simulink model "TEST_2"  (R2024a)
settings: Solver=VariableStepAuto  StartTime=0.0  StopTime=1  RelTol=1e-3
values from neighbouring files (symbols this model uses):
  a = 1.3    [TEST.m]    (also in batter_y.m = -k_omega / J)
  autoRecharge = 0    [TEST.m]
  Cdc = 278e-3    (= 0.278)    [TEST.m]    (also in batter_y.m)
  Efficiency = 96    [TEST.m]
  fg = 60    [TEST.m]    (also in batter_y.m)
  Fn = 60    [TEST.m]
  Gn = 1000    [TEST.m]    (also in batter_y.m)
  Initial_kWh_pc = 80    [TEST.m]
  Ipv_n = Isc_n*(Rp+Rs)/Rp    (= 8.21426513558)    [TEST.m]    (also in batter_y.m)
  Isc_n = 8.21    [TEST.m]    (also in batter_y.m)
  k = 1.3806503e-23    [TEST.m]    (also in batter_y.m)
  KI = 0.0032    [TEST.m]    (also in batter_y.m)
  Ki_C = Rc/tau_C    (= 0.768)    [TEST.m]    (also in batter_y.m)
  Ki_DC = omega_DC^2*Cdc    [TEST.m]    (also in batter_y.m)
  Ki_P = 1/(Ki_pq*tau_P)    [TEST.m]    (also in batter_y.m)
  Ki_PLL = Kp_PLL/tau_PLL    [TEST.m]    (also in batter_y.m)
  Kp_C = Lc/tau_C    (= 0.020372)    [TEST.m]    (also in batter_y.m)
  Kp_DC = 2*xi_DC*omega_DC*Cdc    [TEST.m]    (also in batter_y.m)
  Kp_P = tau_C/(Ki_pq*tau_P)    [TEST.m]    (also in batter_y.m)
  Kp_PLL = xi_PLL*2*omega_PLL/Vp    [TEST.m]    (also in batter_y.m)
  KV = -0.123    [TEST.m]    (also in batter_y.m)
  KVmp = Vmp_n/Voc_n    (= 0.799392097264)    [TEST.m]    (also in batter_y.m)
  kWh_Rated = 100    [TEST.m]
  Lc = 20.372e-6    (= 2.0372e-05)    [TEST.m]    (also in batter_y.m)
  LowChrgLim = LimitVec(2)    [TEST.m]
  Np = 345    [TEST.m]    (also in batter_y.m)
  Ns = 45    [TEST.m]    (also in batter_y.m)
  Ns_cell = 54    [TEST.m]    (also in batter_y.m)
  Pnom = PnomkW*1e3    (= 500000)    [TEST.m]    (also in batter_y.m = 1500000)
  Precharge = 50    [TEST.m]
  q = 1.6021764e-19    [TEST.m]    (also in batter_y.m)
  Rc = 0.768e-3    (= 0.000768)    [TEST.m]    (also in batter_y.m)
  RechargeSOC = 11    [TEST.m]
  Rp = 425.405    [TEST.m]    (also in batter_y.m)
  Rs = 0.221    [TEST.m]    (also in batter_y.m)
  Tn = 25    [TEST.m]    (also in batter_y.m)
  UpChrgLim = LimitVec(1)    [TEST.m]
  Vdc = 1200    [TEST.m]    (also in batter_y.m)
  Vn = 4000    [TEST.m]
  Voc_n = 32.9    [TEST.m]    (also in batter_y.m)
  Vp = Ug*sqrt(2)/sqrt(3)    [TEST.m]    (also in batter_y.m)
libraries: spsSeriesRLCBranchLib x21, spsThreePhaseSeriesRLCLoadLib x7, simulink x6, spsSeriesRLCLoadLib x5, spsGroundLib x5, slpidlib x5, spsControlledVoltageSourceLib x3, spsThreePhaseVIMeasurementLib x2, spsCurrentMeasurementLib x2, spsControlledCurrentSourceLib x2, spsThreePhaseTransformerTwoWindingsLib x2, spsThreePhaseSourceLib x1
(part 1 of 2)
settings Model: Creator=Dell  LastModifiedBy=Dell

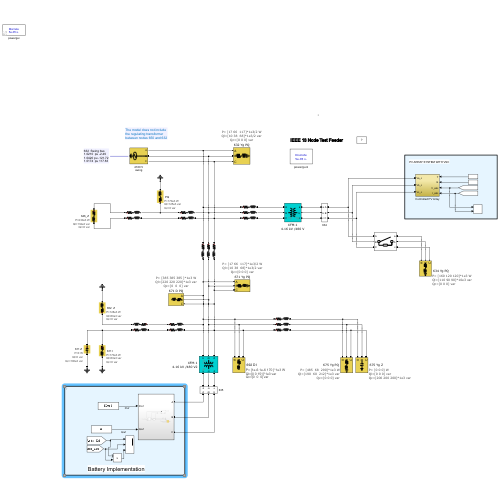
[thumbnail: Simulink's stored preview of the top-level diagram]
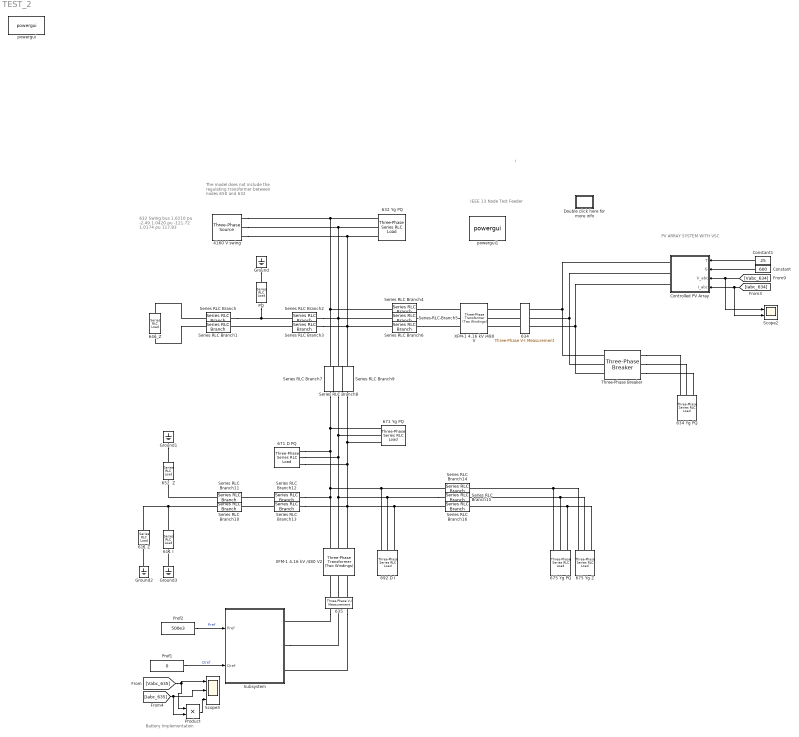
== system TEST_2 ==
  note: PV ARRAY SYSTEM WITH VSC
  note: 632 Swing bus
      | 1.0210 pu -2.49
      | 1.0420 pu -121.72
      | 1.0174 pu 117.83
  note: The model does not include
      | the regulating transformer
      | between nodes 650 and 632
  note: IEEE 13 Node Test Feeder
  note: i
  note: Battery Implementation
  " 634 Yg PQ " : spsThreePhaseSeriesRLCLoadLib/Three-Phase Series RLC Load  LConnTagsString=A|B|C  Configuration=Y (grounded)  NominalVoltage=120e3  Vabc=[ 0.993805 1.0218 0.995862]*277.128  Vabcp=[1e3 1e3 1e3]  NominalFrequency=60  UnbalancedPower=on  ActivePower=1e+006  InductivePower=0  CapacitivePower=0  Pabc=[160 120 120]*1e3  QLabc=[110 90 90]*10e3  QCabc=[0 0 0]  Pabcp=[10e3 9e3 11e3]  QLabcp=[100 90 110]  QCabcp=[100 90 110]  Measurements=None  LoadType=constant PQ
      settings: AttributesFormatString=|
      | P= %<Pabc> W
      | Ql=%<QLabc> var
      | Qc=%<QCabc> var
  4160 V swing : spsThreePhaseSourceLib/Three-Phase Source  InternalConnection=Yg  VoltagePhases=on  Voltage=4.16e3  PhaseAngle=0  Voltage_phases=[ 1.021 1.042 1.0174]*2401.78  PhaseAngles_phases=[ -2.49 -121.72 117.83]  Frequency=60  NonIdealSource=off  SpecifyImpedance=on  Resistance=0.8929  Inductance=16.58e-3  ShortCircuitLevel=100e6  BaseVoltage=120e3  XRratio=10  BusType=swing  Pref=0  Qref=0  Prefabc=[0 0 0]  Qrefabc=[0 0 0]  Qmin="[-inf  -inf -inf]"  Qmax="[inf  inf inf]"
  611 I : spsSeriesRLCLoadLib/Series RLC Load  LConnTagsString=a  RConnTagsString=__new0  NominalVoltage=0.986941*2401.78  NominalFrequency=60  ActivePower=170e3  InductivePower=80e3  CapacitivePower=0  Setx0=off  InitialVoltage=0  SetiL0=off  InitialCurrent=0  Measurements=Branch voltage and current  LoadType=constant I
      settings: AttributesFormatString=|
      | P=%<ActivePower> W
      | Ql=%<InductivePower> var
      | Qc=%<CapacitivePower> var
  611 Z : spsSeriesRLCLoadLib/Series RLC Load  LConnTagsString=a  RConnTagsString=__new0  NominalVoltage=4160/sqrt(3)  NominalFrequency=60  ActivePower=0  InductivePower=0  CapacitivePower=100e3  Setx0=off  InitialVoltage=0  SetiL0=off  InitialCurrent=0  Measurements=None  LoadType=constant Z
      settings: AttributesFormatString=|
      | P=%<ActivePower> W
      | Ql=%<InductivePower> var
      | Qc=%<CapacitivePower> var
  632 Yg PQ : spsThreePhaseSeriesRLCLoadLib/Three-Phase Series RLC Load  LConnTagsString=A|B|C  Configuration=Y (grounded)  NominalVoltage=120e3  Vabc=[ 1.021 1.042 1.0174]*2401.78  Vabcp=[1e3 1e3 1e3]  NominalFrequency=60  UnbalancedPower=on  ActivePower=1e+006  InductivePower=0  CapacitivePower=0  Pabc="[17 66  117]*1e3/2"  QLabc="[10 38  68]*1e3/2"  QCabc=[0 0 0]  Pabcp=[10e3 9e3 11e3]  QLabcp=[100 90 110]  QCabcp=[100 90 110]  Measurements=None  LoadType=constant PQ
      settings: AttributesFormatString=|
      | P= %<Pabc> W
      | Ql=%<QLabc> var
      | Qc=%<QCabc> var
  634 : spsThreePhaseVIMeasurementLib/Three-Phase V-I Measurement  VoltageMeasurement=phase-to-ground  SetLabelV=on  LabelV=Vabc_634  Vpu=off  VpuLL=off  CurrentMeasurement=yes  SetLabelI=on  LabelI=Iabc_634  Ipu=off  Pbase=100e6  Vbase=4160  OutputType=Complex  PhasorSimulation=off  PSBequivalent=0
  635 : spsThreePhaseVIMeasurementLib/Three-Phase V-I Measurement  VoltageMeasurement=phase-to-ground  SetLabelV=on  LabelV=Vabc_635  Vpu=off  VpuLL=off  CurrentMeasurement=yes  SetLabelI=on  LabelI=Iabc_635  Ipu=off  Pbase=100e6  Vbase=4160  OutputType=Complex  PhasorSimulation=off  PSBequivalent=0
  646_Z : spsSeriesRLCLoadLib/Series RLC Load  LConnTagsString=a  RConnTagsString=__new0  NominalVoltage=4160  NominalFrequency=60  ActivePower=230e3  InductivePower=132e3  CapacitivePower=0  Setx0=off  InitialVoltage=0  SetiL0=off  InitialCurrent=0  Measurements=None  LoadType=constant Z
      settings: AttributesFormatString=|
      | P=%<ActivePower> W
      | Ql=%<InductivePower> var
      | Qc=%<CapacitivePower> var
  "652  Z " : spsSeriesRLCLoadLib/Series RLC Load  LConnTagsString=a  RConnTagsString=__new0  NominalVoltage=4160/sqrt(3)  NominalFrequency=60  ActivePower=128e3  InductivePower=86e3  CapacitivePower=0  Setx0=off  InitialVoltage=0  SetiL0=off  InitialCurrent=0  Measurements=None  LoadType=constant Z
      settings: AttributesFormatString=|
      | P=%<ActivePower> W
      | Ql=%<InductivePower> var
      | Qc=%<CapacitivePower> var
  671 D PQ : spsThreePhaseSeriesRLCLoadLib/Three-Phase Series RLC Load  LConnTagsString=A|B|C  Configuration=Delta  NominalVoltage=120e3  Vabc="[1  1  1]*120e3/sqrt(3)"  Vabcp=[ 1.73773 1.77224 1.71484]*2401.78  NominalFrequency=60  UnbalancedPower=on  ActivePower=1e+006  InductivePower=0  CapacitivePower=0  Pabc="[17 66  117]*1e3/2"  QLabc="[10 38  68]*1e3/2"  QCabc=[0 0 0]  Pabcp=[385 385 385 ]*1e3  QLabcp=[220 220 220]*1e3  QCabcp="[0  0  0]"  Measurements=Branch voltages and currents  LoadType=constant PQ
      settings: AttributesFormatString=|
      | P= %<Pabcp> W
      | Ql=%<QLabcp> var
      | Qc=%<QCabcp> var
  671 Yg PQ : spsThreePhaseSeriesRLCLoadLib/Three-Phase Series RLC Load  LConnTagsString=A|B|C  Configuration=Y (grounded)  NominalVoltage=120e3  Vabc=[ 0.987076 1.0519 0.978043]*2401.78  Vabcp=[1e3 1e3 1e3]  NominalFrequency=60  UnbalancedPower=on  ActivePower=1e+006  InductivePower=0  CapacitivePower=0  Pabc="[17 66  117]*1e3/2"  QLabc="[10 38  68]*1e3/2"  QCabc=[0 0 0]  Pabcp=[10e3 9e3 11e3]  QLabcp=[100 90 110]  QCabcp=[100 90 110]  Measurements=None  LoadType=constant PQ
      settings: AttributesFormatString=|
      | P= %<Pabc> W
      | Ql=%<QLabc> var
      | Qc=%<QCabc> var
  675 Yg PQ : spsThreePhaseSeriesRLCLoadLib/Three-Phase Series RLC Load  LConnTagsString=A|B|C  Configuration=Y (grounded)  NominalVoltage=120e3  Vabc=[ 0.98063 1.05431 0.975983]*2401.78  Vabcp=[1e3 1e3 1e3]  NominalFrequency=60  UnbalancedPower=on  ActivePower=1e+006  InductivePower=0  CapacitivePower=0  Pabc="[485  68  290]*1e3"  QLabc="[190  60  212]*1e3"  QCabc=[0 0 0]  Pabcp=[10e3 9e3 11e3]  QLabcp=[100 90 110]  QCabcp=[100 90 110]  Measurements=Branch voltages and currents  LoadType=constant PQ
      settings: AttributesFormatString=|
      | P= %<Pabc> W
      | Ql=%<QLabc> var
      | Qc=%<QCabc> var
  675 Yg Z : spsThreePhaseSeriesRLCLoadLib/Three-Phase Series RLC Load  LConnTagsString=A|B|C  Configuration=Y (grounded)  NominalVoltage=120e3  Vabc="[1  1  1]*4160/sqrt(3)"  Vabcp=[1e3 1e3 1e3]  NominalFrequency=60  UnbalancedPower=on  ActivePower=1e+006  InductivePower=0  CapacitivePower=0  Pabc=[0 0 0]  QLabc=[0 0 0]  QCabc=[200 200 200]*1e3  Pabcp=[10e3 9e3 11e3]  QLabcp=[100 90 110]  QCabcp=[100 90 110]  Measurements=None  LoadType=constant Z
      settings: AttributesFormatString=|
      | P= %<Pabc> W
      | Ql=%<QLabc> var
      | Qc=%<QCabc> var
  692 D I : spsThreePhaseSeriesRLCLoadLib/Three-Phase Series RLC Load  LConnTagsString=A|B|C  Configuration=Delta  NominalVoltage=120e3  Vabc="[1  1  1]*120e3/sqrt(3)"  Vabcp=[ 1.73488 1.75203 1.72341]*2401.78  NominalFrequency=60  UnbalancedPower=on  ActivePower=1e+006  InductivePower=0  CapacitivePower=0  Pabc="[17 66  117]*1e3/2"  QLabc="[10 38  68]*1e3/2"  QCabc=[0 0 0]  Pabcp=[1e-6 1e-6 170 ]*1e3  QLabcp=[0 0 151]*1e3  QCabcp="[0  0  0]"  Measurements=Branch voltages and currents  LoadType=constant I
      settings: AttributesFormatString=|
      | P= %<Pabcp> W
      | Ql=%<QLabcp> var
      | Qc=%<QCabcp> var
  Constant : Constant  Value=600
  Constant1 : Constant  Value=25
  Controlled PV Array : Subsystem
      settings: PortSchema="{\"entries\":[{\"content\":{\"sides\":[{\"content\":{\"connectorIds\":[\"LConn1\",\"LConn2\",\"LConn3\"]},\"type\":\"ConnectorPlacement.EquallySpacedRectSide\",\"uuid\":\"92a05cf9-a19b-475d-bffb-9406018f82f4\"},{\"content\":{\"connectorIds\":[\"In1\",\"In2\",\"In3\",\"In4\"],\"side\":\"RIGHT\"},\"type\":\"ConnectorPlacement.EquallySpacedRectSide\",\"uuid\":\"83076eb6-0a86-49d7-8932-035501cdc6f6\"},{\"content\":{\"side\":\"TOP\"},\"type\":\"ConnectorPlacement.EquallySpacedRectSide\",\"uuid\":\"ba2310df-ee07-4a5c-88ff-ef0f81658322\"}]},\"type\":\"ConnectorPlacement.EquallySpacedConnector\",\"uuid\":\"9e64c472-0dae-4bb4-8eb3-3329c328d412\"}],\"packageUris\":[\"http://schema.mathworks.com/mf0/Connector/R2020b\"],\"version\":\"1.0\"}"
  Double click here for more info : Subsystem
      settings: OpenFcn=showdemo(bdroot(gcb))
      mask Display: disp('?')
  Ground{,1..3} (4 alike) : spsGroundLib/Ground  LConnTagsString=a
  PQ : spsSeriesRLCLoadLib/Series RLC Load  LConnTagsString=a  RConnTagsString=__new0  NominalVoltage=1.03289*2401.78  NominalFrequency=60  ActivePower=170e3  InductivePower=125e3  CapacitivePower=0  Setx0=off  InitialVoltage=0  SetiL0=off  InitialCurrent=0  Measurements=None  LoadType=constant PQ
      settings: AttributesFormatString=|
      | P=%<ActivePower> W
      | Ql=%<InductivePower> var
      | Qc=%<CapacitivePower> var
  Pref1 : Constant  Value=0
  Pref2 : Constant  Value=500e3
  Product : Product
  Scope2 : Scope  NumInputPorts=2
  Scope3 : Scope  NumInputPorts=3
  Series RLC Branch : spsSeriesRLCBranchLib/Series RLC Branch  LConnTagsString=__new0  RConnTagsString=__new0  BranchType=RL  Resistance=0.07553  Inductance=0.20302e-3  SetiL0=off  InitialCurrent=0  Capacitance=1e-6  Setx0=off  InitialVoltage=0  Measurements=None
  Series RLC Branch1 : spsSeriesRLCBranchLib/Series RLC Branch  LConnTagsString=__new0  RConnTagsString=__new0  BranchType=RL  Resistance=0.07553  Inductance=0.20302e-3  SetiL0=off  InitialCurrent=0  Capacitance=1e-6  Setx0=off  InitialVoltage=0  Measurements=None
  Series RLC Branch10 : spsSeriesRLCBranchLib/Series RLC Branch  LConnTagsString=__new0  RConnTagsString=__new0  BranchType=RL  Resistance=0.07552  Inductance=0.20308e-3  SetiL0=off  InitialCurrent=0  Capacitance=1e-6  Setx0=off  InitialVoltage=0  Measurements=None
  Series RLC Branch11 : spsSeriesRLCBranchLib/Series RLC Branch  LConnTagsString=__new0  RConnTagsString=__new0  BranchType=RL  Resistance=0.20340  Inductance=0.20593e-3  SetiL0=off  InitialCurrent=0  Capacitance=1e-6  Setx0=off  InitialVoltage=0  Measurements=None
  Series RLC Branch12 : spsSeriesRLCBranchLib/Series RLC Branch  LConnTagsString=__new0  RConnTagsString=__new0  BranchType=RL  Resistance=0.07521  Inductance=0.20450e-3  SetiL0=off  InitialCurrent=0  Capacitance=1e-6  Setx0=off  InitialVoltage=0  Measurements=None
  Series RLC Branch13 : spsSeriesRLCBranchLib/Series RLC Branch  LConnTagsString=__new0  RConnTagsString=__new0  BranchType=RL  Resistance=0.07521  Inductance=0.20450e-3  SetiL0=off  InitialCurrent=0  Capacitance=1e-6  Setx0=off  InitialVoltage=0  Measurements=None
  Series RLC Branch14 : spsSeriesRLCBranchLib/Series RLC Branch  LConnTagsString=__new0  RConnTagsString=__new0  BranchType=RL  Resistance=0.07559  Inductance=0.11210e-3  SetiL0=off  InitialCurrent=0  Capacitance=1e-6  Setx0=off  InitialVoltage=0  Measurements=None
  Series RLC Branch15 : spsSeriesRLCBranchLib/Series RLC Branch  LConnTagsString=__new0  RConnTagsString=__new0  BranchType=RL  Resistance=0.07559  Inductance=0.11210e-3  SetiL0=off  InitialCurrent=0  Capacitance=1e-6  Setx0=off  InitialVoltage=0  Measurements=None
  Series RLC Branch16 : spsSeriesRLCBranchLib/Series RLC Branch  LConnTagsString=__new0  RConnTagsString=__new0  BranchType=RL  Resistance=0.07559  Inductance=0.11210e-3  SetiL0=off  InitialCurrent=0  Capacitance=1e-6  Setx0=off  InitialVoltage=0  Measurements=None
  Series RLC Branch2 : spsSeriesRLCBranchLib/Series RLC Branch  LConnTagsString=__new0  RConnTagsString=__new0  BranchType=RL  Resistance=0.12589  Inductance=0.33837e-3  SetiL0=off  InitialCurrent=0  Capacitance=1e-6  Setx0=off  InitialVoltage=0  Measurements=None
  Series RLC Branch3 : spsSeriesRLCBranchLib/Series RLC Branch  LConnTagsString=__new0  RConnTagsString=__new0  BranchType=RL  Resistance=0.12589  Inductance=0.33837e-3  SetiL0=off  InitialCurrent=0  Capacitance=1e-6  Setx0=off  InitialVoltage=0  Measurements=None
  Series RLC Branch4 : spsSeriesRLCBranchLib/Series RLC Branch  LConnTagsString=__new0  RConnTagsString=__new0  BranchType=RL  Resistance=0.07126  Inductance=0.29675e-3  SetiL0=off  InitialCurrent=0  Capacitance=1e-6  Setx0=off  InitialVoltage=0  Measurements=None
  Series RLC Branch5 : spsSeriesRLCBranchLib/Series RLC Branch  LConnTagsString=__new0  RConnTagsString=__new0  BranchType=RL  Resistance=0.07126  Inductance=0.29675e-3  SetiL0=off  InitialCurrent=0  Capacitance=1e-6  Setx0=off  InitialVoltage=0  Measurements=None
  Series RLC Branch6 : spsSeriesRLCBranchLib/Series RLC Branch  LConnTagsString=__new0  RConnTagsString=__new0  BranchType=RL  Resistance=0.07126  Inductance=0.29675e-3  SetiL0=off  InitialCurrent=0  Capacitance=1e-6  Setx0=off  InitialVoltage=0  Measurements=None
  Series RLC Branch7 : spsSeriesRLCBranchLib/Series RLC Branch  LConnTagsString=__new0  RConnTagsString=__new0  BranchType=RL  Resistance=0.13124  Inductance=1.03632e-3  SetiL0=off  InitialCurrent=0  Capacitance=1e-6  Setx0=off  InitialVoltage=0  Measurements=None
  Series RLC Branch8 : spsSeriesRLCBranchLib/Series RLC Branch  LConnTagsString=__new0  RConnTagsString=__new0  BranchType=RL  Resistance=0.13124  Inductance=1.03632e-3  SetiL0=off  InitialCurrent=0  Capacitance=1e-6  Setx0=off  InitialVoltage=0  Measurements=None
  Series RLC Branch9 : spsSeriesRLCBranchLib/Series RLC Branch  LConnTagsString=__new0  RConnTagsString=__new0  BranchType=RL  Resistance=0.13124  Inductance=1.03632e-3  SetiL0=off  InitialCurrent=0  Capacitance=1e-6  Setx0=off  InitialVoltage=0  Measurements=None
  Subsystem : Subsystem
  Three-Phase Breaker : spsThreePhaseBreakerLib/Three-Phase Breaker  InitialState=open  SwitchA=on  SwitchB=on  SwitchC=on  SwitchTimes=0.3  External=off  BreakerResistance=0.01  SnubberResistance=1e6  SnubberCapacitance=inf  Measurements=None
  XFM-1 4.16 kV /480 V : spsThreePhaseTransformerTwoWindingsLib/Three-Phase Transformer (Two Windings)  Winding1Connection=Yg  Winding2Connection=Yg  CoreType=Three single-phase transformers  SetSaturation=off  Hysteresis=off  DataFile='hysteresis'  SetInitialFlux=off  Measurements=None  UNITS=pu  NominalPower=[ 500e3 , 60 ]  Winding1=[4160 0.011 0.02]  Winding2=[480 0 0]  Rm=500  Lm=500  L0=0.5  Saturation=[0 0;0.0024 1.2;1 1.52]  InitialFluxes=[0.8 -0.8 0.7]  BreakLoop=off  DiscreteSolver=Trapezoidal iterative  DataType=off  TransfoNumber=1
  XFM-1 4.16 kV /480 V2 : spsThreePhaseTransformerTwoWindingsLib/Three-Phase Transformer (Two Windings)  Winding1Connection=Yg  Winding2Connection=Yg  CoreType=Three single-phase transformers  SetSaturation=off  Hysteresis=off  DataFile='hysteresis'  SetInitialFlux=off  Measurements=None  UNITS=pu  NominalPower=[ 500e3 , 60 ]  Winding1=[4160 0.011 0.02]  Winding2=[480 0 0]  Rm=500  Lm=500  L0=0.5  Saturation=[0 0;0.0024 1.2;1 1.52]  InitialFluxes=[0.8 -0.8 0.7]  BreakLoop=off  DiscreteSolver=Trapezoidal iterative  DataType=off  TransfoNumber=1
  powergui : sps_lib/powergui  Priority=1  SimulationMode=Discrete  SampleTime=50e-6  frequency=60  Iterations=50  frequencyindice=0  Pbase=100e6  ErrMax=1e-4  UnitsV=kV  UnitsW=MW  buscounter=0  FunctionMessages=off  echomessages=off  EnableUseOfTLC=off  CurrentSourceSwitches=off  DisableSnubberDevices=off  DisableRonSwitches=off  DisableVfSwitches=off  DisplayEquations=off  AutomaticDiscreteSolvers=off  SolverType=Tustin/Backward Euler (TBE)  Interpol=off  ExternalGateDelay=off  methode=off  Ts=100  x0status=blocks  SPID=on  SwTol=0  HookPort=off  NonlinearTolerance=1e-4  nMaxIteration=100  ContinueOnMaxIteration=off  RestoreLinks=warning  ResistiveCurrentMeasurement=off  Frange=[0:2:500]  Ylog=off  Xlog=on  ShowGrid=off  save=off  variable=ZData  structure=0  ZoomFFT=off  StartTime=0.0  cycles=1  DisplayStyle=1  fundamental=60  FreqAxis=off  MaxFrequency=1000  frequencyindicesteady=1  RmsSteady=1  display=off
  powergui1 : spspowerguiLib/powergui  Priority=1  SimulationMode=Discrete  SampleTime=5e-5  frequency=60  Iterations=50  frequencyindice=0  Pbase=100e3  ErrMax=0.0001  UnitsV=kV  UnitsW=kW  buscounter=0  FunctionMessages=off  echomessages=off  EnableUseOfTLC=off  CurrentSourceSwitches=off  DisableSnubberDevices=off  DisableRonSwitches=off  DisableVfSwitches=off  DisplayEquations=off  AutomaticDiscreteSolvers=off  SolverType=Tustin/Backward Euler (TBE)  Interpol=off  ExternalGateDelay=off  methode=off  Ts=0  x0status=blocks  SPID=off  SwTol=0  HookPort=off  NonlinearTolerance=1e-4  nMaxIteration=100  ContinueOnMaxIteration=off  RestoreLinks=warning  ResistiveCurrentMeasurement=off  Frange=[0:2:500]  Ylog=off  Xlog=on  ShowGrid=off  save=off  variable=ZData  structure=0  ZoomFFT=on  StartTime=0.0  cycles=1  DisplayStyle=1  fundamental=60  FreqAxis=off  MaxFrequency=1000  frequencyindicesteady=1  RmsSteady=1  display=off
  wires:
  [Iabc_634] -> Scope2/2, Controlled PV Array/4(I_abc)
  Pref2/1 -> Subsystem/1(Pref)  "Pref"
  [Iabc_635] -> Product/2, Scope3/2
  [Vabc_634] -> Scope2/1, Controlled PV Array/3(V_abc)
  [Vabc_635] -> Product/1, Scope3/1
  Constant/1 -> Controlled PV Array/2(G)
  Pref1/1 -> Subsystem/2(Qref)  "Qref"
  Constant1/1 -> Controlled PV Array/1(T)
  Product/1 -> Scope3/3
  connections:
  Series RLC Branch5/LConn1 -- Series RLC Branch2/RConn1 -- 632 Yg PQ/LConn2 -- 4160 V swing/RConn2 -- Series RLC Branch8/LConn1
  XFM-1 4.16 kV /480 V2/LConn3 -- Series RLC Branch12/RConn1 -- 692 D I/LConn1 -- Series RLC Branch14/LConn1 -- 671 D PQ/LConn1 -- Series RLC Branch7/RConn1 -- 671 Yg PQ/LConn1
  Series RLC Branch2/LConn1 -- Series RLC Branch/RConn1 -- PQ/LConn1
  675 Yg PQ/LConn1 -- Series RLC Branch14/RConn1 -- 675 Yg Z/LConn1
  Three-Phase Breaker/LConn2 -- 634/LConn2 -- Controlled PV Array/LConn2
  Series RLC Branch6/LConn1 -- Series RLC Branch3/RConn1 -- 632 Yg PQ/LConn3 -- 4160 V swing/RConn3 -- Series RLC Branch9/LConn1
  675 Yg PQ/LConn3 -- Series RLC Branch16/RConn1 -- 675 Yg Z/LConn3
  Series RLC Branch15/LConn1 -- 671 D PQ/LConn2 -- Series RLC Branch8/RConn1 -- 671 Yg PQ/LConn2 -- XFM-1 4.16 kV /480 V2/LConn2 -- 692 D I/LConn2
  675 Yg PQ/LConn2 -- Series RLC Branch15/RConn1 -- 675 Yg Z/LConn2
  671 Yg PQ/LConn3 -- Series RLC Branch9/RConn1 -- Series RLC Branch13/RConn1 -- XFM-1 4.16 kV /480 V2/LConn1 -- 692 D I/LConn3 -- Series RLC Branch16/LConn1 -- 671 D PQ/LConn3
  Three-Phase Breaker/LConn3 -- 634/LConn3 -- Controlled PV Array/LConn3
  4160 V swing/RConn1 -- 632 Yg PQ/LConn1 -- Series RLC Branch4/LConn1 -- Series RLC Branch7/LConn1
  Series RLC Branch10/LConn1 -- 611 Z/LConn1 -- 611 I/LConn1
  Three-Phase Breaker/LConn1 -- 634/LConn1 -- Controlled PV Array/LConn1
  635/LConn3 -- Subsystem/RConn3
  Subsystem/RConn2 -- 635/LConn2
  Series RLC Branch3/LConn1 -- Series RLC Branch1/RConn1
  Ground/LConn1 -- PQ/RConn1
  Series RLC Branch11/RConn1 -- "652  Z "/LConn1
  635/LConn1 -- Subsystem/RConn1
  Series RLC Branch1/LConn1 -- 646_Z/RConn1
  Ground3/LConn1 -- 611 I/RConn1
  634/RConn1 -- XFM-1 4.16 kV /480 V/RConn1
  Ground2/LConn1 -- 611 Z/RConn1
  634/RConn2 -- XFM-1 4.16 kV /480 V/RConn2
  Series RLC Branch/LConn1 -- 646_Z/LConn1
  Ground1/LConn1 -- "652  Z "/RConn1
  635/RConn1 -- XFM-1 4.16 kV /480 V2/RConn3
  Series RLC Branch12/LConn1 -- Series RLC Branch11/LConn1
  Series RLC Branch5/RConn1 -- XFM-1 4.16 kV /480 V/LConn2
  XFM-1 4.16 kV /480 V/LConn3 -- Series RLC Branch6/RConn1
  635/RConn3 -- XFM-1 4.16 kV /480 V2/RConn1
  Three-Phase Breaker/RConn2 -- " 634 Yg PQ "/LConn2
  635/RConn2 -- XFM-1 4.16 kV /480 V2/RConn2
  634/RConn3 -- XFM-1 4.16 kV /480 V/RConn3
  XFM-1 4.16 kV /480 V/LConn1 -- Series RLC Branch4/RConn1
  Three-Phase Breaker/RConn3 -- " 634 Yg PQ "/LConn3
  Three-Phase Breaker/RConn1 -- " 634 Yg PQ "/LConn1
  Series RLC Branch13/LConn1 -- Series RLC Branch10/RConn1

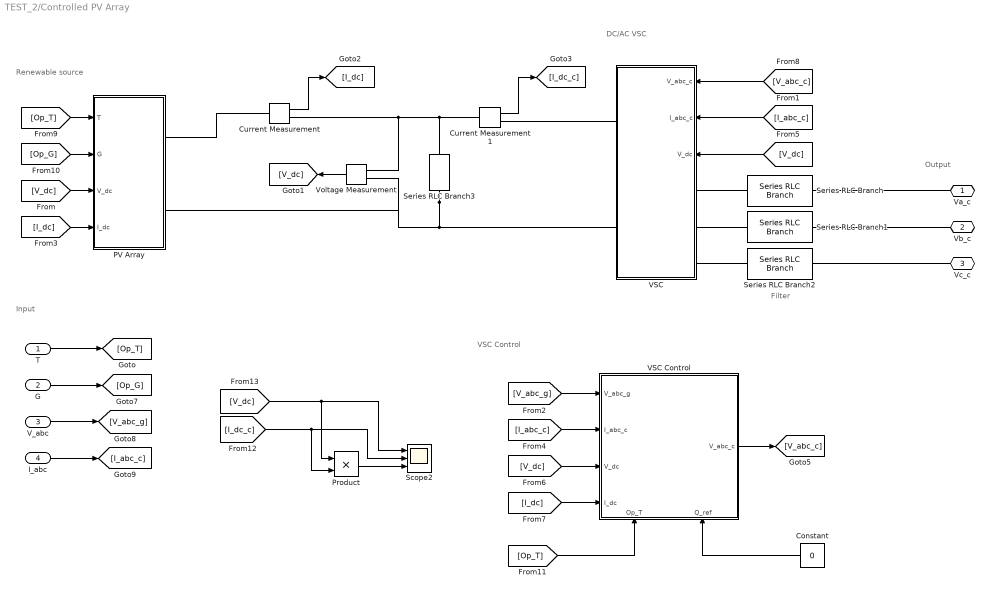
== system TEST_2/Controlled PV Array ==
  note: Output
  note: Input
  note: Filter
  note: Renewable source
  note: VSC Control
  note: DC/AC VSC
  T : Inport
  G : Inport  Port=2
  V_abc : Inport  Port=3
  I_abc : Inport  Port=4
  Constant : Constant  Value=0
  Current Measurement : spsCurrentMeasurementLib/Current Measurement  PhasorSimulation=off  OutputType=Complex  PSBequivalent=0
  Current Measurement1 : spsCurrentMeasurementLib/Current Measurement  PhasorSimulation=off  OutputType=Complex  PSBequivalent=0
  PV Array : Subsystem
  Product : Product
  Scope2 : Scope  NumInputPorts=3
  Series RLC Branch : spsSeriesRLCBranchLib/Series RLC Branch  LConnTagsString=__new0  RConnTagsString=__new0  BranchType=RL  Resistance=Rc  Inductance=Lc  SetiL0=off  InitialCurrent=0  Capacitance=1e-6  Setx0=off  InitialVoltage=0  Measurements=None
  Series RLC Branch1 : spsSeriesRLCBranchLib/Series RLC Branch  LConnTagsString=__new0  RConnTagsString=__new0  BranchType=RL  Resistance=Rc  Inductance=Lc  SetiL0=off  InitialCurrent=0  Capacitance=1e-6  Setx0=off  InitialVoltage=0  Measurements=None
  Series RLC Branch2 : spsSeriesRLCBranchLib/Series RLC Branch  LConnTagsString=__new0  RConnTagsString=__new0  BranchType=RL  Resistance=Rc  Inductance=Lc  SetiL0=off  InitialCurrent=0  Capacitance=1e-6  Setx0=off  InitialVoltage=0  Measurements=None
  Series RLC Branch3 : spsSeriesRLCBranchLib/Series RLC Branch  LConnTagsString=__new0  RConnTagsString=__new0  BranchType=C  Resistance=0.3  Inductance=1e-3  SetiL0=off  InitialCurrent=0  Capacitance=Cdc  Setx0=on  InitialVoltage=Vdc  Measurements=None
  VSC : Subsystem
  VSC Control : Subsystem
      settings: PortSchema="{\"entries\":[{\"content\":{\"sides\":[{\"content\":{\"connectorIds\":[\"In1\",\"In2\",\"In3\",\"In4\"]},\"type\":\"ConnectorPlacement.EquallySpacedRectSide\",\"uuid\":\"1f0c866f-1355-4493-8a8b-fecd52da2e06\"},{\"content\":{\"connectorIds\":[\"Out1\"],\"side\":\"RIGHT\"},\"type\":\"ConnectorPlacement.EquallySpacedRectSide\",\"uuid\":\"e0482316-46fe-491c-835b-46d73fa6817a\"},{\"content\":{\"side\":\"TOP\"},\"type\":\"ConnectorPlacement.EquallySpacedRectSide\",\"uuid\":\"b85aba4d-c629-42a9-b30e-3179992b26cb\"},{\"content\":{\"connectorIds\":[\"In5\",\"In6\"],\"side\":\"BOTTOM\"},\"type\":\"ConnectorPlacement.EquallySpacedRectSide\",\"uuid\":\"2c79aeba-fb98-4b17-8331-d72a75796cf8\"}]},\"type\":\"ConnectorPlacement.EquallySpacedConnector\",\"uuid\":\"5586ce08-6872-4275-b1b0-323c6fc0897a\"}],\"packageUris\":[\"http://schema.mathworks.com/mf0/Connector/R2020b\"],\"version\":\"1.0\"}"
  Voltage Measurement : spsVoltageMeasurementLib/Voltage Measurement  PhasorSimulation=off  OutputType=Complex  PSBequivalent=0
  Va_c : PMIOPort  Side=Left
  Vb_c : PMIOPort  Port=2  Side=Left
  Vc_c : PMIOPort  Port=3  Side=Left
  wires:
  [V_abc_c] -> VSC/1(V_abc_c)
  Constant/1 -> VSC Control/6(Q_ref)
  I_abc/1 -> [I_abc_c]
  Current Measurement1/1 -> [I_dc_c]
  [V_dc] -> Scope2/1, Product/1
  [I_dc_c] -> Scope2/2, Product/2
  [I_dc] -> VSC Control/4(I_dc)
  Voltage Measurement/1 -> [V_dc]
  [V_abc_g] -> VSC Control/1(V_abc_g)
  VSC Control/1(V_abc_c) -> [V_abc_c]
  [V_dc] -> PV Array/3(V_dc)
  Current Measurement/1 -> [I_dc]
  Product/1 -> Scope2/3
  [Op_T] -> VSC Control/5(Op_T)
  [V_dc] -> VSC/3(V_dc)
  V_abc/1 -> [V_abc_g]
  [Op_T] -> PV Array/1(T)
  [V_dc] -> VSC Control/3(V_dc)
  [Op_G] -> PV Array/2(G)
  [I_abc_c] -> VSC Control/2(I_abc_c)
  [I_abc_c] -> VSC/2(I_abc_c)
  [I_dc] -> PV Array/4(I_dc)
  G/1 -> [Op_G]
  T/1 -> [Op_T]
  connections:
  VSC/LConn2 -- Series RLC Branch1/RConn1
  Series RLC Branch3/RConn1 -- Voltage Measurement/LConn2 -- PV Array/RConn2 -- VSC/RConn2
  Current Measurement1/LConn1 -- Series RLC Branch3/LConn1 -- Current Measurement/RConn1 -- Voltage Measurement/LConn1
  PV Array/RConn1 -- Current Measurement/LConn1
  VSC/LConn1 -- Series RLC Branch/RConn1
  VSC/LConn3 -- Series RLC Branch2/RConn1
  Va_c/RConn1 -- Series RLC Branch/LConn1
  VSC/RConn1 -- Current Measurement1/RConn1
  Vc_c/RConn1 -- Series RLC Branch2/LConn1
  Vb_c/RConn1 -- Series RLC Branch1/LConn1

== system TEST_2/Double click here for more info ==

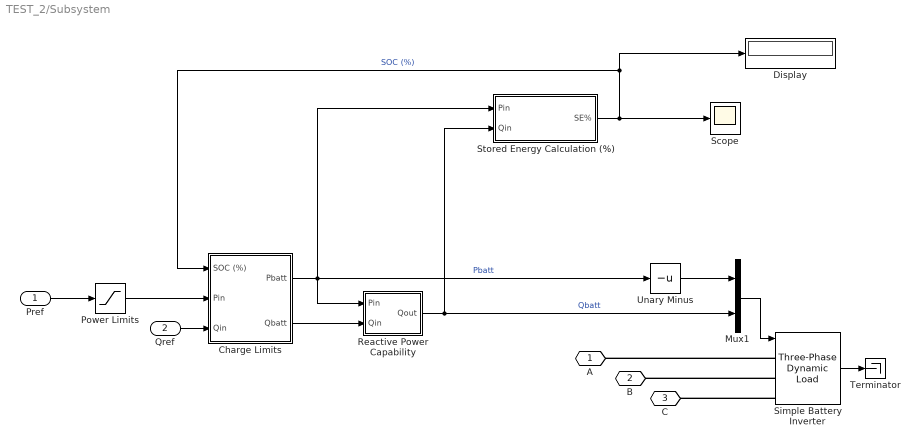
== system TEST_2/Subsystem ==
  Pref : Inport
  Qref : Inport  Port=2
  Charge Limits : Subsystem
  Display : Display
  Mux1 : Mux  Inputs=2
  Power Limits : Saturate  UpperLimit=Pnom  LowerLimit=-Pnom
  Reactive Power Capability : Subsystem
  Scope : Scope
  Simple Battery Inverter : spsThreePhaseDynamicLoadLib/Three-Phase Dynamic Load  NominalVoltage=[Vn Fn]  ActiveReactivePowers=[-500000 -3.38813e-13]  PositiveSequence=[0.999844 -0.0038635]  ExternalControl=on  NpNq=[1.3 2]  TimeConstants="[0  0  0  0]"  MinimumVoltage=0.7  Tfilter=1e-2  LoadFlowParameters=[4,0,0,0,0]
  Stored Energy Calculation (%) : Subsystem
  Terminator : Terminator
  Unary Minus : UnaryMinus
  A : PMIOPort  Side=Right
  B : PMIOPort  Port=2  Side=Right
  C : PMIOPort  Port=3  Side=Right
  wires:
  Qref/1 -> Charge Limits/3(Qin)
  Power Limits/1 -> Charge Limits/2(Pin)
  Stored Energy Calculation (%)/1(SE%) -> Display/1, Charge Limits/1(SOC (%)), Scope/1  "SOC (%)"
  Pref/1 -> Power Limits/1
  Charge Limits/1(Pbatt) -> Reactive Power Capability/1(Pin), Unary Minus/1, Stored Energy Calculation (%)/1(Pin)  "Pbatt"
  Reactive Power Capability/1(Qout) -> Mux1/2, Stored Energy Calculation (%)/2(Qin)  "Qbatt"
  Mux1/1 -> Simple Battery Inverter/1
  Charge Limits/2(Qbatt) -> Reactive Power Capability/2(Qin)
  Simple Battery Inverter/1 -> Terminator/1
  Unary Minus/1 -> Mux1/1
  connections:
  Simple Battery Inverter/LConn1 -- A/RConn1
  Simple Battery Inverter/LConn2 -- B/RConn1
  Simple Battery Inverter/LConn3 -- C/RConn1

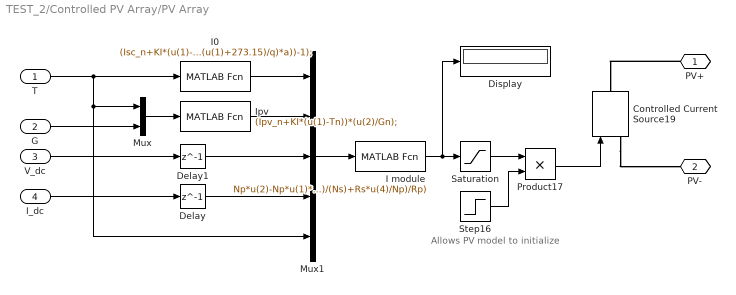
== system TEST_2/Controlled PV Array/PV Array ==
  note: Allows PV model to initialize
  T : Inport
  G : Inport  Port=2
  V_dc : Inport  Port=3
  I_dc : Inport  Port=4
  Controlled Current Source19 : spsControlledCurrentSourceLib/Controlled Current Source  Initialize=on  Source_Type=AC  Amplitude=0  Phase=0  Frequency=0  Measurements=None
  Delay : Delay  DelayLength=1  InitialCondition=1000
  Delay1 : Delay  DelayLength=1  InitialCondition=1200
  Display : Display
  I module : MATLABFcn  MATLABFcn=Np*u(2)-Np*u(1)*(exp((u(3)/(Ns)+Rs*u(4)/Np)/((Ns_cell*k*(u(5)+273.15)/q)*a))-1)-Np*((u(3)/(Ns)+Rs*u(4)/Np)/Rp)  OutputDimensions=1
  I0 : MATLABFcn  MATLABFcn=(Isc_n+KI*(u(1)-Tn))/(exp((Voc_n+KV*(u(1)-Tn))/((Ns_cell*k*(u(1)+273.15)/q)*a))-1);  OutputDimensions=1
  Ipv : MATLABFcn  MATLABFcn=(Ipv_n+KI*(u(1)-Tn))*(u(2)/Gn);  OutputDimensions=1
  Mux : Mux  Inputs=2
  Mux1 : Mux  Inputs=5
  Product17 : Product
  Saturation : Saturate  UpperLimit=10e6  LowerLimit=0.1
  Step16 : Step  Time=0.001  SampleTime=0
  PV+ : PMIOPort  Side=Right
  PV- : PMIOPort  Port=2  Side=Right
  wires:
  Mux1/1 -> I module/1
  G/1 -> Mux/2
  Mux/1 -> Ipv/1
  T/1 -> Mux1/5, Mux/1, I0/1
  Ipv/1 -> Mux1/2
  I0/1 -> Mux1/1
  Delay/1 -> Mux1/4
  I_dc/1 -> Delay/1
  Saturation/1 -> Product17/1
  Step16/1 -> Product17/2
  Product17/1 -> Controlled Current Source19/1
  Delay1/1 -> Mux1/3
  V_dc/1 -> Delay1/1
  I module/1 -> Display/1, Saturation/1
  connections:
  PV+/RConn1 -- Controlled Current Source19/RConn1
  Controlled Current Source19/LConn1 -- PV-/RConn1

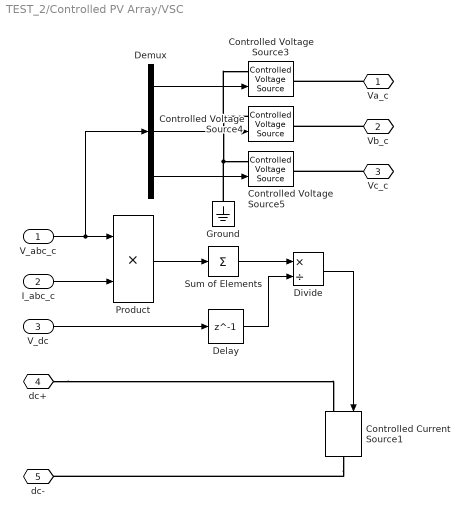
== system TEST_2/Controlled PV Array/VSC ==
  V_abc_c : Inport
  I_abc_c : Inport  Port=2
  V_dc : Inport  Port=3
  Controlled Current Source1 : spsControlledCurrentSourceLib/Controlled Current Source  Initialize=on  Source_Type=AC  Amplitude=0  Phase=0  Frequency=0  Measurements=None
  Controlled Voltage Source3 : spsControlledVoltageSourceLib/Controlled Voltage Source  Initialize=off  Source_Type=AC  Amplitude=0  Phase=0  Frequency=60  Measurements=None
  Controlled Voltage Source4 : spsControlledVoltageSourceLib/Controlled Voltage Source  Initialize=off  Source_Type=AC  Amplitude=0  Phase=0  Frequency=60  Measurements=None
  Controlled Voltage Source5 : spsControlledVoltageSourceLib/Controlled Voltage Source  Initialize=off  Source_Type=AC  Amplitude=0  Phase=0  Frequency=60  Measurements=None
  Delay : Delay  DelayLength=1  InitialCondition=1200
  Demux : Demux  Outputs=3
  Divide : Product  Inputs=*/  RndMeth=Zero  SaturateOnIntegerOverflow=on
  Ground : spsGroundLib/Ground  LConnTagsString=a
  Product : Product
  Sum of Elements : Sum  Inputs=+
  Va_c : PMIOPort  Side=Left
  Vb_c : PMIOPort  Port=2  Side=Left
  Vc_c : PMIOPort  Port=3  Side=Left
  dc+ : PMIOPort  Port=4  Side=Right
  dc- : PMIOPort  Port=5  Side=Right
  wires:
  Product/1 -> Sum of Elements/1
  I_abc_c/1 -> Product/2
  V_abc_c/1 -> Demux/1, Product/1
  Demux/2 -> Controlled Voltage Source4/1
  Demux/1 -> Controlled Voltage Source3/1
  Demux/3 -> Controlled Voltage Source5/1
  Sum of Elements/1 -> Divide/1
  Divide/1 -> Controlled Current Source1/1
  V_dc/1 -> Delay/1
  Delay/1 -> Divide/2
  connections:
  Vb_c/RConn1 -- Controlled Voltage Source4/RConn1
  Va_c/RConn1 -- Controlled Voltage Source3/RConn1
  Controlled Voltage Source4/LConn1 -- Controlled Voltage Source3/LConn1 -- Controlled Voltage Source5/LConn1 -- Ground/LConn1
  Vc_c/RConn1 -- Controlled Voltage Source5/RConn1
  Controlled Current Source1/RConn1 -- dc-/RConn1
  dc+/RConn1 -- Controlled Current Source1/LConn1

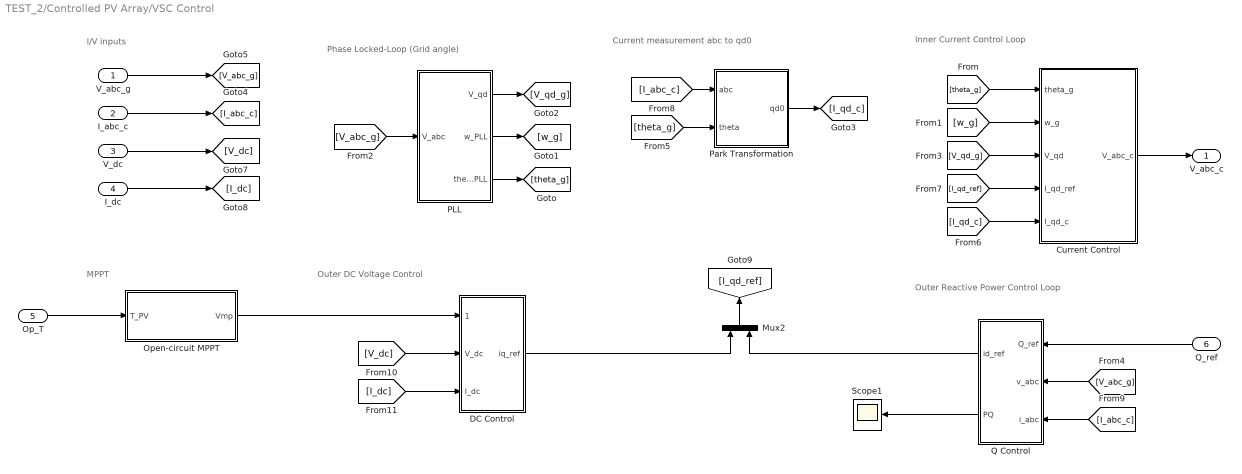
== system TEST_2/Controlled PV Array/VSC Control ==
  note: I/V inputs
  note: Phase Locked-Loop (Grid angle)
  note: Current measurement abc to qd0
  note: Inner Current Control Loop
  note: Outer Reactive Power Control Loop
  note: MPPT
  note: Outer DC Voltage Control
  V_abc_g : Inport
  I_abc_c : Inport  Port=2
  V_dc : Inport  Port=3
  I_dc : Inport  Port=4
  Op_T : Inport  Port=5
  Q_ref : Inport  Port=6
  Current Control : Subsystem
  DC Control : Subsystem
  Mux2 : Mux  Inputs=2
  Open-circuit MPPT : Subsystem
  PLL : Subsystem
  Park Transformation : Subsystem
  Q Control : Subsystem
  Scope1 : Scope
  V_abc_c : Outport
  wires:
  Park Transformation/1(qd0) -> [I_qd_c]
  [theta_g] -> Current Control/1(theta_g)
  PLL/3(theta_PLL) -> [theta_g]
  [I_qd_ref] -> Current Control/4(I_qd_ref)
  [theta_g] -> Park Transformation/2(theta)
  PLL/1(V_qd) -> [V_qd_g]
  PLL/2(w_PLL) -> [w_g]
  [w_g] -> Current Control/2(w_g)
  [V_qd_g] -> Current Control/3(V_qd)
  [I_qd_c] -> Current Control/5(I_qd_c)
  Current Control/1(V_abc_c) -> V_abc_c/1
  [V_abc_g] -> Q Control/2(v_abc)
  [I_abc_c] -> Q Control/3(i_abc)
  [V_dc] -> DC Control/2(V_dc)
  [I_dc] -> DC Control/3(I_dc)
  [I_abc_c] -> Park Transformation/1(abc)
  V_dc/1 -> [V_dc]
  I_abc_c/1 -> [I_abc_c]
  V_abc_g/1 -> [V_abc_g]
  I_dc/1 -> [I_dc]
  DC Control/1(iq_ref) -> Mux2/1
  Q Control/1(id_ref) -> Mux2/2
  Mux2/1 -> [I_qd_ref]
  Q_ref/1 -> Q Control/1(Q_ref)
  Op_T/1 -> Open-circuit MPPT/1(T_PV)
  Q Control/2(PQ) -> Scope1/1
  Open-circuit MPPT/1(Vmp) -> DC Control/1(V_dc_ref)
  [V_abc_g] -> PLL/1(V_abc)

== system TEST_2/Subsystem/Charge Limits ==
  SOC (%) : Inport
  Pin : Inport  Port=2
  Qin : Inport  Port=3
  Overcharge Check : Subsystem
  Undercharge Check : Subsystem
  Pbatt : Outport  VectorParamsAs1DForOutWhenUnconnected=off
  Qbatt : Outport  Port=2  VectorParamsAs1DForOutWhenUnconnected=off
  wires:
  SOC (%)/1 -> Overcharge Check/1(SOC (%)), Undercharge Check/1(SOC (%))
  Undercharge Check/2(Qout) -> Qbatt/1
  Pin/1 -> Overcharge Check/2(Pin)
  Overcharge Check/1(Pout) -> Undercharge Check/2(Pin)
  Qin/1 -> Overcharge Check/3(Qin)
  Undercharge Check/1(Pout) -> Pbatt/1  "Pbatt"
  Overcharge Check/2(Qout) -> Undercharge Check/3(Qin)

== system TEST_2/Subsystem/Reactive Power Capability ==
  Pin : Inport
  Qin : Inport  Port=2
  Constant : Constant  Value=Pnom
  Math Function : Math  Operator=square  SignedPower=on
  Math Function1 : Math  Operator=square  SignedPower=on
  Saturation Dynamic : simulink/Discontinuities/Saturation Dynamic  OutMin=[]  OutMax=[]  OutDataTypeStr=Inherit: Same as second input  OutDataType=fixdt(1, 16)  OutScaling=2^-10  DoSatur=off
  Sqrt : Sqrt
  Sum : Sum  Inputs=-+|
  Unary Minus : UnaryMinus
  Qout : Outport  VectorParamsAs1DForOutWhenUnconnected=off
  wires:
  Sqrt/1 -> Saturation Dynamic/1, Unary Minus/1
  Math Function1/1 -> Sum/1
  Math Function/1 -> Sum/2
  Constant/1 -> Math Function/1
  Sum/1 -> Sqrt/1
  Unary Minus/1 -> Saturation Dynamic/3
  Saturation Dynamic/1 -> Qout/1
  Pin/1 -> Math Function1/1
  Qin/1 -> Saturation Dynamic/2

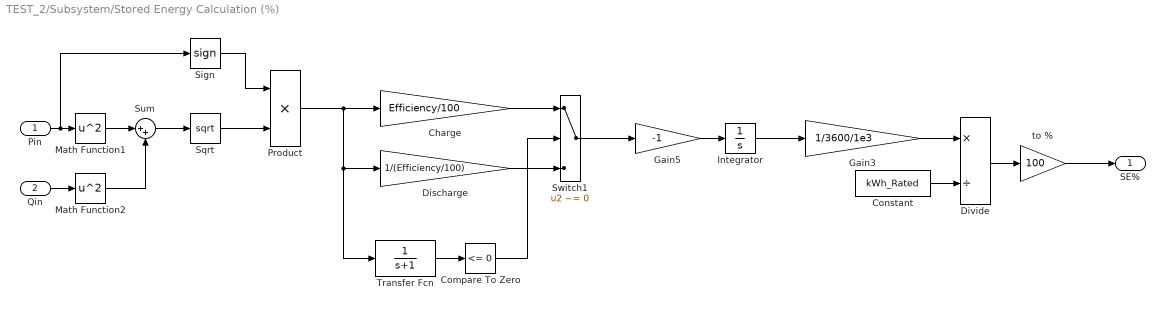
== system TEST_2/Subsystem/Stored Energy Calculation (%) ==
  Pin : Inport
  Qin : Inport  Port=2
  Charge : Gain  Gain=Efficiency/100
  Compare To Zero : simulink/Logic and Bit Operations/Compare To Zero  relop=<=  OutDataTypeStr=boolean
  Constant : Constant  Value=kWh_Rated
  Discharge : Gain  Gain=1/(Efficiency/100)
  Divide : Product  Inputs=*/
  Gain3 : Gain  Gain=1/3600/1e3
  Gain5 : Gain  Gain=-1
  Integrator : Integrator  InitialCondition=(Initial_kWh_pc/100)*kWh_Rated*3600*1e3
  Math Function1 : Math  Operator=square  SignedPower=on
  Math Function2 : Math  Operator=square  SignedPower=on
  Product : Product
  Sign : Signum
  Sqrt : Sqrt
  Sum : Sum  Inputs=|++
  Switch1 : Switch  Criteria=u2 ~= 0  SaturateOnIntegerOverflow=off  InputSameDT=off
  Transfer Fcn : TransferFcn  Denominator=[1 1]
  to % : Gain  Gain=100
  SE% : Outport  VectorParamsAs1DForOutWhenUnconnected=off
  wires:
  Sign/1 -> Product/1
  Sqrt/1 -> Product/2
  Sum/1 -> Sqrt/1
  Math Function2/1 -> Sum/2
  Math Function1/1 -> Sum/1
  Qin/1 -> Math Function2/1
  Pin/1 -> Math Function1/1, Sign/1
  Product/1 -> Transfer Fcn/1, Discharge/1, Charge/1
  Discharge/1 -> Switch1/3
  Gain5/1 -> Integrator/1
  to %/1 -> SE%/1
  Transfer Fcn/1 -> Compare To Zero/1
  Switch1/1 -> Gain5/1
  Gain3/1 -> Divide/1
  Constant/1 -> Divide/2
  Charge/1 -> Switch1/1
  Divide/1 -> to %/1
  Compare To Zero/1 -> Switch1/2
  Integrator/1 -> Gain3/1

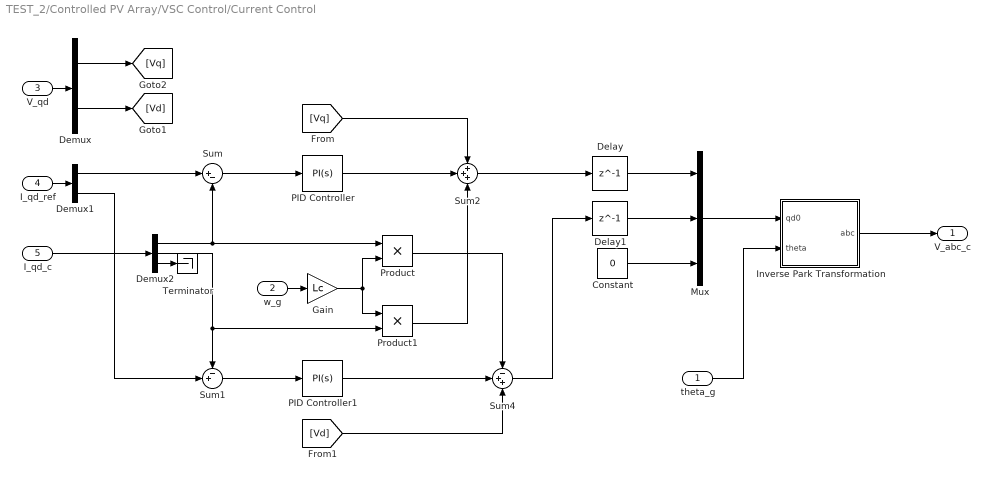
== system TEST_2/Controlled PV Array/VSC Control/Current Control ==
  theta_g : Inport
  w_g : Inport  Port=2
  V_qd : Inport  Port=3
  I_qd_ref : Inport  Port=4
  I_qd_c : Inport  Port=5
  Constant : Constant  Value=0
  Delay : Delay  DelayLength=1  InitialCondition=0.1
  Delay1 : Delay  DelayLength=1  InitialCondition=0.1
  Demux : Demux  Outputs=2
  Demux1 : Demux  Outputs=2
  Demux2 : Demux  Outputs=3
  Gain : Gain  Gain=Lc
  Inverse Park Transformation : Subsystem
  Mux : Mux  Inputs=3
  PID Controller : slpidlib/PID Controller  Controller=PI  Form=Parallel  TimeDomain=Continuous-time  UseExternalTs=off  SampleTime=-1  IntegratorMethod=Forward Euler  FilterMethod=Forward Euler  ControllerParametersSource=internal  P=Kp_C  I=Ki_C  UseKiTs=off  D=0  UseExternalDerivativeSource=off  N=100  UseFilter=on  TunerSelectOption=Transfer Function Based (PID Tuner App)  InitialConditionSource=internal  InitialConditionForIntegrator=0  InitialConditionForFilter=0  DifferentiatorICPrevScaledInput=0  ExternalReset=none  TrackingMode=off  Kt=1  LimitOutput=off  SatLimitsSource=internal  UpperSaturationLimit=inf  LowerSaturationLimit=-inf  LinearizeAsGain=on  AntiWindupMode=none  Kb=1  LimitIntegrator=off  UpperIntegratorSaturationLimit=inf  LowerIntegratorSaturationLimit=-inf  POutMin=[]  POutMax=[]  IOutMin=[]  IOutMax=[]  DOutMin=[]  DOutMax=[]  NOutMin=[]  NOutMax=[]  SumOutMin=[]  SumOutMax=[]  SaturationOutMin=[]  SaturationOutMax=[]  PParamMin=[]  PParamMax=[]  IParamMin=[]  IParamMax=[]  DParamMin=[]  DParamMax=[]  NParamMin=[]  NParamMax=[]  KbParamMin=[]  KbParamMax=[]  KtParamMin=[]  KtParamMax=[]  KbOutMin=[]  KbOutMax=[]  KtOutMin=[]  KtOutMax=[]  IntegratorOutMin=[]  IntegratorOutMax=[]  FilterOutMin=[]  FilterOutMax=[]  SumI1OutMin=[]  SumI1OutMax=[]  SumI2OutMin=[]  SumI2OutMax=[]  SumI3OutMin=[]  SumI3OutMax=[]  SumI4OutMin=[]  SumI4OutMax=[]  SumDOutMin=[]  SumDOutMax=[]  DifferentiatorOutMin=[]  DifferentiatorOutMax=[]  FilterDiffOutCoefMin=[]  FilterDiffOutCoefMax=[]  ReciprocalOutMin=[]  ReciprocalOutMax=[]  SumDenOutMin=[]  SumDenOutMax=[]  SumNumOutMin=[]  SumNumOutMax=[]  DivideOutMin=[]  DivideOutMax=[]  UdiffTsProdOutMin=[]  UdiffTsProdOutMax=[]  NTsProdOutMin=[]  NTsProdOutMax=[]  UintegralTsProdOutMin=[]  UintegralTsProdOutMax=[]  UngainTsProdOutMin=[]  UngainTsProdOutMax=[]  ClampingZeroOutDataTypeStr=Inherit: Inherit via back propagation  ClampingZeroOutMin=[]  ClampingZeroOutMax=[]  FilterDenConstantOutDataTypeStr=Inherit: Inherit via back propagation  FilterDenConstantOutMin=[]  FilterDenConstantOutMax=[]  PCopyOutDataTypeStr=Inherit: Inherit via back propagation  PCopyOutMin=[]  PCopyOutMax=[]  NCopyOutDataTypeStr=Inherit: Inherit via back propagation  NCopyOutMin=[]  NCopyOutMax=[]  IntegratorContinuousStateAttributes=''  IntegratorStateMustResolveToSignalObject=off  IntegratorRTWStateStorageClass=Auto  FilterContinuousStateAttributes=''  FilterStateMustResolveToSignalObject=off  FilterRTWStateStorageClass=Auto  ParallelPVariant=InternalParameters  IdealPVariant=Disabled  IVariant=InternalParameters  DVariant=Disabled  IntegratorVariant=Continuous  SatVariant=Disabled  AWVariant=Passthrough  PCopyVariant=Disabled  TRVariant=Disabled  FdbkBlocksVariant=Forward  IdealPFdbkVariant=Disabled  SatFdbkVariant=Disabled  DerivativeFilterVariant=Disabled  NVariant=Disabled  NCopyVariant=Disabled_SignalSpec  FilterICVariant=Disabled  IntegratorICVariant=InternalICs  ExternalResetVariant=Disabled  TRSumVariant=Passthrough  SumFdbkVariant=Disabled  SumVariant=Sum_PI  TsampFilterVariant=InternalTs  TsampNgainVariant=Passthrough  TsampIntegralVariant=Disabled_SignalSpec  ExternalSaturationOutDataTypeStr=Inherit: Same as second input  DerivativeSourceVariant=Disabled
  PID Controller1 : slpidlib/PID Controller  Controller=PI  Form=Parallel  TimeDomain=Continuous-time  UseExternalTs=off  SampleTime=-1  IntegratorMethod=Forward Euler  FilterMethod=Forward Euler  ControllerParametersSource=internal  P=Kp_C  I=Ki_C  UseKiTs=off  D=0  UseExternalDerivativeSource=off  N=100  UseFilter=on  TunerSelectOption=Transfer Function Based (PID Tuner App)  InitialConditionSource=internal  InitialConditionForIntegrator=0  InitialConditionForFilter=0  DifferentiatorICPrevScaledInput=0  ExternalReset=none  TrackingMode=off  Kt=1  LimitOutput=off  SatLimitsSource=internal  UpperSaturationLimit=inf  LowerSaturationLimit=-inf  LinearizeAsGain=on  AntiWindupMode=none  Kb=1  LimitIntegrator=off  UpperIntegratorSaturationLimit=inf  LowerIntegratorSaturationLimit=-inf  POutMin=[]  POutMax=[]  IOutMin=[]  IOutMax=[]  DOutMin=[]  DOutMax=[]  NOutMin=[]  NOutMax=[]  SumOutMin=[]  SumOutMax=[]  SaturationOutMin=[]  SaturationOutMax=[]  PParamMin=[]  PParamMax=[]  IParamMin=[]  IParamMax=[]  DParamMin=[]  DParamMax=[]  NParamMin=[]  NParamMax=[]  KbParamMin=[]  KbParamMax=[]  KtParamMin=[]  KtParamMax=[]  KbOutMin=[]  KbOutMax=[]  KtOutMin=[]  KtOutMax=[]  IntegratorOutMin=[]  IntegratorOutMax=[]  FilterOutMin=[]  FilterOutMax=[]  SumI1OutMin=[]  SumI1OutMax=[]  SumI2OutMin=[]  SumI2OutMax=[]  SumI3OutMin=[]  SumI3OutMax=[]  SumI4OutMin=[]  SumI4OutMax=[]  SumDOutMin=[]  SumDOutMax=[]  DifferentiatorOutMin=[]  DifferentiatorOutMax=[]  FilterDiffOutCoefMin=[]  FilterDiffOutCoefMax=[]  ReciprocalOutMin=[]  ReciprocalOutMax=[]  SumDenOutMin=[]  SumDenOutMax=[]  SumNumOutMin=[]  SumNumOutMax=[]  DivideOutMin=[]  DivideOutMax=[]  UdiffTsProdOutMin=[]  UdiffTsProdOutMax=[]  NTsProdOutMin=[]  NTsProdOutMax=[]  UintegralTsProdOutMin=[]  UintegralTsProdOutMax=[]  UngainTsProdOutMin=[]  UngainTsProdOutMax=[]  ClampingZeroOutDataTypeStr=Inherit: Inherit via back propagation  ClampingZeroOutMin=[]  ClampingZeroOutMax=[]  FilterDenConstantOutDataTypeStr=Inherit: Inherit via back propagation  FilterDenConstantOutMin=[]  FilterDenConstantOutMax=[]  PCopyOutDataTypeStr=Inherit: Inherit via back propagation  PCopyOutMin=[]  PCopyOutMax=[]  NCopyOutDataTypeStr=Inherit: Inherit via back propagation  NCopyOutMin=[]  NCopyOutMax=[]  IntegratorContinuousStateAttributes=''  IntegratorStateMustResolveToSignalObject=off  IntegratorRTWStateStorageClass=Auto  FilterContinuousStateAttributes=''  FilterStateMustResolveToSignalObject=off  FilterRTWStateStorageClass=Auto  ParallelPVariant=InternalParameters  IdealPVariant=Disabled  IVariant=InternalParameters  DVariant=Disabled  IntegratorVariant=Continuous  SatVariant=Disabled  AWVariant=Passthrough  PCopyVariant=Disabled  TRVariant=Disabled  FdbkBlocksVariant=Forward  IdealPFdbkVariant=Disabled  SatFdbkVariant=Disabled  DerivativeFilterVariant=Disabled  NVariant=Disabled  NCopyVariant=Disabled_SignalSpec  FilterICVariant=Disabled  IntegratorICVariant=InternalICs  ExternalResetVariant=Disabled  TRSumVariant=Passthrough  SumFdbkVariant=Disabled  SumVariant=Sum_PI  TsampFilterVariant=InternalTs  TsampNgainVariant=Passthrough  TsampIntegralVariant=Disabled_SignalSpec  ExternalSaturationOutDataTypeStr=Inherit: Same as second input  DerivativeSourceVariant=Disabled
  Product : Product
  Product1 : Product
  Sum : Sum  Inputs=|+-
  Sum1 : Sum  Inputs=-+|
  Sum2 : Sum  Inputs=+++
  Sum4 : Sum  Inputs=-++
  Terminator : Terminator
  V_abc_c : Outport
  wires:
  Demux2/2 -> Product1/2, Sum1/1
  V_qd/1 -> Demux/1
  Sum1/1 -> PID Controller1/1
  Sum/1 -> PID Controller/1
  Gain/1 -> Product/2, Product1/1
  Demux/2 -> [Vd]
  [Vd] -> Sum4/3
  Mux/1 -> Inverse Park Transformation/1(qd0)
  Constant/1 -> Mux/3
  Demux1/1 -> Sum/1
  Demux2/1 -> Sum/2, Product/1
  theta_g/1 -> Inverse Park Transformation/2(theta)
  Demux/1 -> [Vq]
  PID Controller/1 -> Sum2/2
  PID Controller1/1 -> Sum4/2
  Product1/1 -> Sum2/3
  [Vq] -> Sum2/1
  Inverse Park Transformation/1(abc) -> V_abc_c/1
  Product/1 -> Sum4/1
  Demux1/2 -> Sum1/2
  w_g/1 -> Gain/1
  I_qd_ref/1 -> Demux1/1
  I_qd_c/1 -> Demux2/1
  Demux2/3 -> Terminator/1
  Sum2/1 -> Delay/1
  Delay/1 -> Mux/1
  Delay1/1 -> Mux/2
  Sum4/1 -> Delay1/1

== system TEST_2/Controlled PV Array/VSC Control/DC Control ==
  V_dc_ref : Inport
  V_dc : Inport  Port=2
  I_dc : Inport  Port=3
  Gain : Gain
  Gain1 : Gain  Gain=-1
  Gain2 : Gain  Gain=(2/3)*(Vdc/Vp)
  PID Controller : slpidlib/PID Controller  Controller=PI  Form=Parallel  TimeDomain=Continuous-time  UseExternalTs=off  SampleTime=-1  IntegratorMethod=Forward Euler  FilterMethod=Forward Euler  ControllerParametersSource=internal  P=Kp_DC  I=Ki_DC  UseKiTs=off  D=0  UseExternalDerivativeSource=off  N=100  UseFilter=on  TunerSelectOption=Transfer Function Based (PID Tuner App)  InitialConditionSource=internal  InitialConditionForIntegrator=0  InitialConditionForFilter=0  DifferentiatorICPrevScaledInput=0  ExternalReset=none  TrackingMode=off  Kt=1  LimitOutput=off  SatLimitsSource=internal  UpperSaturationLimit=inf  LowerSaturationLimit=-inf  LinearizeAsGain=on  AntiWindupMode=none  Kb=1  LimitIntegrator=off  UpperIntegratorSaturationLimit=inf  LowerIntegratorSaturationLimit=-inf  POutMin=[]  POutMax=[]  IOutMin=[]  IOutMax=[]  DOutMin=[]  DOutMax=[]  NOutMin=[]  NOutMax=[]  SumOutMin=[]  SumOutMax=[]  SaturationOutMin=[]  SaturationOutMax=[]  PParamMin=[]  PParamMax=[]  IParamMin=[]  IParamMax=[]  DParamMin=[]  DParamMax=[]  NParamMin=[]  NParamMax=[]  KbParamMin=[]  KbParamMax=[]  KtParamMin=[]  KtParamMax=[]  KbOutMin=[]  KbOutMax=[]  KtOutMin=[]  KtOutMax=[]  IntegratorOutMin=[]  IntegratorOutMax=[]  FilterOutMin=[]  FilterOutMax=[]  SumI1OutMin=[]  SumI1OutMax=[]  SumI2OutMin=[]  SumI2OutMax=[]  SumI3OutMin=[]  SumI3OutMax=[]  SumI4OutMin=[]  SumI4OutMax=[]  SumDOutMin=[]  SumDOutMax=[]  DifferentiatorOutMin=[]  DifferentiatorOutMax=[]  FilterDiffOutCoefMin=[]  FilterDiffOutCoefMax=[]  ReciprocalOutMin=[]  ReciprocalOutMax=[]  SumDenOutMin=[]  SumDenOutMax=[]  SumNumOutMin=[]  SumNumOutMax=[]  DivideOutMin=[]  DivideOutMax=[]  UdiffTsProdOutMin=[]  UdiffTsProdOutMax=[]  NTsProdOutMin=[]  NTsProdOutMax=[]  UintegralTsProdOutMin=[]  UintegralTsProdOutMax=[]  UngainTsProdOutMin=[]  UngainTsProdOutMax=[]  ClampingZeroOutDataTypeStr=Inherit: Inherit via back propagation  ClampingZeroOutMin=[]  ClampingZeroOutMax=[]  FilterDenConstantOutDataTypeStr=Inherit: Inherit via back propagation  FilterDenConstantOutMin=[]  FilterDenConstantOutMax=[]  PCopyOutDataTypeStr=Inherit: Inherit via back propagation  PCopyOutMin=[]  PCopyOutMax=[]  NCopyOutDataTypeStr=Inherit: Inherit via back propagation  NCopyOutMin=[]  NCopyOutMax=[]  IntegratorContinuousStateAttributes=''  IntegratorStateMustResolveToSignalObject=off  IntegratorRTWStateStorageClass=Auto  FilterContinuousStateAttributes=''  FilterStateMustResolveToSignalObject=off  FilterRTWStateStorageClass=Auto  ParallelPVariant=InternalParameters  IdealPVariant=Disabled  IVariant=InternalParameters  DVariant=Disabled  IntegratorVariant=Continuous  SatVariant=Disabled  AWVariant=Passthrough  PCopyVariant=Disabled  TRVariant=Disabled  FdbkBlocksVariant=Forward  IdealPFdbkVariant=Disabled  SatFdbkVariant=Disabled  DerivativeFilterVariant=Disabled  NVariant=Disabled  NCopyVariant=Disabled_SignalSpec  FilterICVariant=Disabled  IntegratorICVariant=InternalICs  ExternalResetVariant=Disabled  TRSumVariant=Passthrough  SumFdbkVariant=Disabled  SumVariant=Sum_PI  TsampFilterVariant=InternalTs  TsampNgainVariant=Passthrough  TsampIntegralVariant=Disabled_SignalSpec  ExternalSaturationOutDataTypeStr=Inherit: Same as second input  DerivativeSourceVariant=Disabled
  Sum : Sum  Inputs=|+-
  Sum1 : Sum  Inputs=|+-
  iq_ref : Outport
  wires:
  V_dc/1 -> Sum/2
  Sum1/1 -> Gain1/1
  Sum/1 -> PID Controller/1
  I_dc/1 -> Gain/1
  Gain1/1 -> Gain2/1
  Gain2/1 -> iq_ref/1
  Gain/1 -> Sum1/2
  V_dc_ref/1 -> Sum/1
  PID Controller/1 -> Sum1/1

== system TEST_2/Controlled PV Array/VSC Control/Open-circuit MPPT ==
  T_PV : Inport
  Constant3 : Constant  Value=Tn
  Constant4 : Constant  Value=Voc_n
  Gain : Gain  Gain=KV
  Gain1 : Gain  Gain=KVmp
  Gain2 : Gain  Gain=Ns
  Sum : Sum  Inputs=|++
  Sum1 : Sum  Inputs=|+-
  Vmp : Outport
  wires:
  Gain/1 -> Sum/1
  Constant4/1 -> Sum/2
  Sum/1 -> Gain1/1
  T_PV/1 -> Sum1/1
  Sum1/1 -> Gain/1
  Gain1/1 -> Gain2/1
  Gain2/1 -> Vmp/1
  Constant3/1 -> Sum1/2
